simulink model "SimV8"  (R2024b)
settings: Solver=FixedStepAuto  StartTime=0.0  StopTime=10  RelTol=1e-3
model workspace (MAT data in the model file):
  Sig = Simulink.Signal
  Sig.Dimensions = -1
  Sig.DimensionsMode = 'auto'
  Sig.Complexity = 'auto'
  Sig.SampleTime = -1
  Sig.SamplingMode = 'auto'
  Sig.DataType = 'auto'
values from neighbouring files (symbols this model uses):
  CanaryAmplitude = 0.25    [ConfigData.sldd]
  CanaryCarrierFrequency = 20000.0    [ConfigData.sldd]
  CanaryDataRate = 100.0    [ConfigData.sldd]
  DataAmplitude = 0.1    [ConfigData.sldd]
  FmDecoderFrameSize = 128.0    [ConfigData.sldd]
  FmFrequencyDifferential = 400.0    [ConfigData.sldd]
  PreConvolveDownsample = 32.0    [ConfigData.sldd]
  SampleRate = 48000.0    [ConfigData.sldd]
  WalshCodeLength = 16.0    [ConfigData.sldd]
undefined symbols (not defined in the file or in its folder): FmFrequencyDataCache, ModulatedCanaryCachedCycle, WalshCodeCache
libraries: dspstat3 x4, simulink x3, dspfdesign x3, dspsnks4 x2, audiosources x2, commchan3 x1
settings Model: DataDictionary=ConfigData.sldd  PauseTimes=4.5  PacingRate=0.007100  Creator=calum  LastModifiedBy=calum
settings SolverCC: AllowMultiTaskInputOutput=on  PositivePriorityOrder=on  AutoInsertRateTranBlk=on
settings OptimizationCC: DefaultParameterBehavior=Inlined  InlineInvariantSignals=on  StateBitsets=on  DataBitsets=on  ZeroExternalMemoryAtStartup=off  ZeroInternalMemoryAtStartup=off  EfficientFloat2IntCast=on  SimCompilerOptimization=on  AccelVerboseBuild=on  MultiThreadedLoops=on
settings DebuggingCC: ReadBeforeWriteMsg=DisableAll  WriteAfterWriteMsg=DisableAll  WriteAfterReadMsg=DisableAll  MultiTaskDSMMsg=none  TasksWithSamePriorityMsg=none  IntegerOverflowMsg=none  IntegerSaturationMsg=none
settings HardwareCC: ProdBitPerLong=64  ProdLongLongMode=on  ProdHWDeviceType=AMD->x86-64 (Linux 64)  TargetBitPerLong=64  TargetBitPerPointer=64  TargetBitPerSizeT=64  TargetBitPerPtrDiffT=64  TargetLargestAtomicFloat=Float  TargetIntDivRoundTo=Zero  TargetEndianess=LittleEndian  TargetWordSize=64  TargetHWDeviceType=Intel->x86-64 (Linux 64)
settings ModelReferenceCC: UpdateModelReferenceTargets=IfOutOfDate  EnableParallelModelReferenceBuilds=on  ParallelModelReferenceMATLABWorkerInit=Copy Base Workspace
settings SFSimCC: SimUserLibraries=/home/calum/.local/matlab/2024b/bin/glnxa64/libmwdsp_halidesim.so  SFSimEcho=off  SimCtrlC=off  SimHardwareAcceleration=native  SimTargetLang=C++
settings RTWCC: GenerateReport=on  RTWUseSimCustomCode=on  CustomLibrary=/home/calum/.local/matlab/2024b/bin/glnxa64/libmwdsp_halidesim.so  BuildConfiguration=Faster Runs  LaunchReport=on  TargetLang=C++  CheckMdlBeforeBuild=Warning
settings CodeAppCC: MaxIdLength=95  MATLABSourceComments=on
settings GRTTargetCC: TargetLangStandard=C++17 (ISO)  MatFileLogging=off  CodeInterfacePackaging=C++ class  OptimizeReductions=on

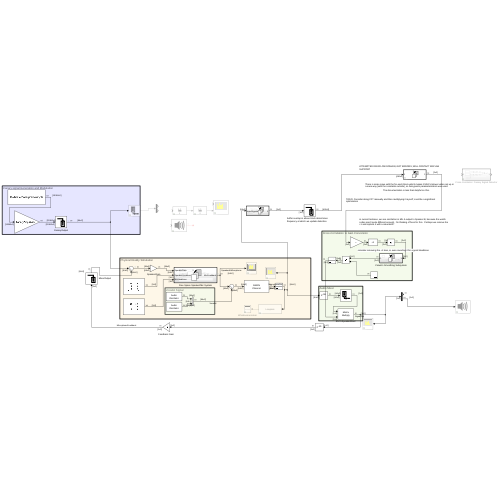
[thumbnail: Simulink's stored preview of the top-level diagram]
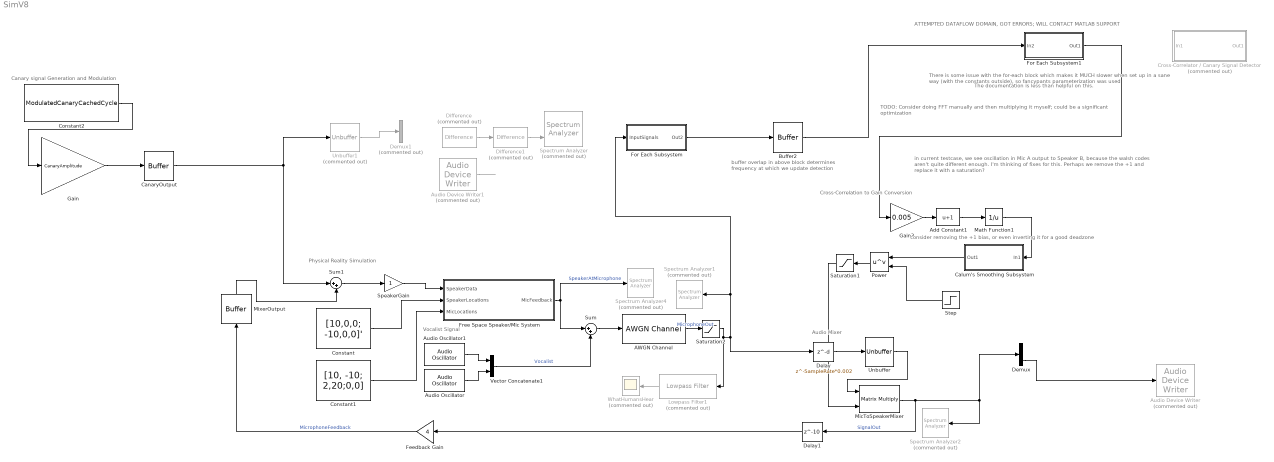
== system SimV8 ==
  note: The documentation is less than helpful on this.
  note: There is some issue with the for-each block which makes it MUCH slower when set up in a sane way (with the constants outside), so fancypants parameterization was used
  note: consider removing the +1 bias, or even inverting it for a good deadzone
  note: in current testcase, we see oscillation in Mic A output to Speaker B, because the walsh codes aren't quite different enough. I'm thinking of fixes for this. Perhaps we remove the +1 and replace it with a saturation?
  note: TODO: Consider doing FFT manually and then multiplying it myself; could be a significant optimization
  note: buffer overlap in above block determines frequency at which we update detection
  note: Canary signal Generation and Modulation
  note: Audio Mixer
  note: Physical Reality Simulation
  note: Vocalist Signal
  note: Cross-Correlation to Gain Conversion
  note: ATTEMPTED DATAFLOW DOMAIN, GOT ERRORS; WILL CONTACT MATLAB SUPPORT
  AWGN Channel : commchan3/AWGN Channel  LegacyMode=off  NoiseMethod="Signal to noise ratio  (SNR)"  noiseMode="Signal to noise ratio  (SNR)"  EbNo=10  EsNo=10  SNR=30  BitsPerSymbol=1  SignalPower=1  SamplesPerSymbol=1  SymbolPeriod=1  VarianceSource=Parameter  Variance=1  RandomStream=Global stream  Seed=67  SimulateUsing=Code generation
  Add Constant1 : Bias  Bias=1  SaturateOnIntegerOverflow=off
  Audio Device Writer : dspsnks4/Audio Device Writer  Commented=on  Driver=ALSA  Device=Default  InheritSampleRate=on  SampleRate=44100  BitDepth=16-bit integer  BufferSize=4096  NumBuffers=10  DefaultOutputChannelMapping=on  OutputChannelMapping=1:2  OutputNumUnderrunSamples=off  DriverIdx=8  DeviceWarnFlag=''
  Audio Device Writer1 : dspsnks4/Audio Device Writer  Commented=on  Driver=ALSA  Device=Default  InheritSampleRate=on  SampleRate=44100  BitDepth=16-bit integer  BufferSize=4096  NumBuffers=10  DefaultOutputChannelMapping=on  OutputChannelMapping=1:2  OutputNumUnderrunSamples=on  DriverIdx=8  DeviceWarnFlag=''
  Audio Oscillator : audiosources/Audio Oscillator  FrequencyPort=off  Frequency=200  AmplitudePort=off  Amplitude=DataAmplitude  DCOffsetPort=off  DCOffset=0  PhaseOffset=0  WidthPort=off  Width=1  DutyCyclePort=off  DutyCycle=0.5  SampsPerFrame=64  Fs=SampleRate  OutputDataType=double  SimulateUsing=Code generation
      settings: SignalType=sine
  Audio Oscillator1 : audiosources/Audio Oscillator  FrequencyPort=off  Frequency=400  AmplitudePort=off  Amplitude=DataAmplitude  DCOffsetPort=off  DCOffset=0  PhaseOffset=0  WidthPort=off  Width=1  DutyCyclePort=off  DutyCycle=0.5  SampsPerFrame=64  Fs=SampleRate  OutputDataType=double  SimulateUsing=Code generation
      settings: SignalType=sine
  Buffer2 : Buffer  N=ceil(SampleRate/32/CanaryDataRate*WalshCodeLength*2)+10  V=ceil(SampleRate/32/CanaryDataRate*WalshCodeLength*2)  OutputFrames=off
  Calum's Smoothing Subsystem : Subsystem  TreatAsAtomicUnit=on
  CanaryOutput : Buffer  OutputFrames=off
  Constant : Constant  Value="[10,0,0;  -10,0,0]'"
  Constant1 : Constant  Value=[10, -10; 2,20;0,0]
  Constant2 : Constant  Value=ModulatedCanaryCachedCycle
  "Cross-Correlator / Canary Signal Detector " : Subsystem  Commented=on  TreatAsAtomicUnit=on
  Delay : Delay  DelayLength=SampleRate*0.002  InitialCondition=0  InputProcessing=Columns as channels (frame based)  UseCircularBuffer=on
  Delay1 : Delay  DelayLength=10  InitialCondition=0  InputProcessing=Columns as channels (frame based)  UseCircularBuffer=on
  Demux : Demux  Outputs=2
  Demux1 : Demux  Commented=on  Outputs=2
  Difference : simulink/Discrete/Difference  Commented=on  ICPrevInput=0.0  OutMin=[]  OutMax=[]  OutDataType=fixdt(1, 16)  OutScaling=2^-10  DoSatur=off
  Difference1 : simulink/Discrete/Difference  Commented=on  ICPrevInput=0.0  OutMin=[]  OutMax=[]  OutDataType=fixdt(1, 16)  OutScaling=2^-10  DoSatur=off
  Feedback Gain : Gain  Gain=4
  For Each Subsystem : Subsystem  TreatAsAtomicUnit=on
  For Each Subsystem1 : Subsystem  TreatAsAtomicUnit=on  mask{CachedCode=WalshCodeCache}
      mask prompts: CachedCode "Walsh Codes"
      settings: RTWSystemCode=Inline
  Free Space Speaker/Mic System : Subsystem  TreatAsAtomicUnit=on
  Gain : Gain  Gain=CanaryAmplitude
  Gain3 : Gain  Gain=0.005
  Lowpass Filter1 : dspfdesign/Lowpass Filter  Commented=on  FilterType=FIR  DesignForMinimumOrder=on  FilterOrder=50  PassbandFrequency=CanaryCarrierFrequency-8000  StopbandFrequency=CanaryCarrierFrequency-1000  PassbandRipple=0.1  StopbandAttenuation=80  SampleRateMode=Specify on dialog  SampleRate=SampleRate  SimulateUsing=Code generation  roundingMode=Floor  coeffsDataTypeStr=fixdt(1,16)
  Math Function1 : Math  Operator=reciprocal
  MicToSpeakerMixer : Product  Multiplication=Matrix(*)
  MixerOutput : Buffer  OutputFrames=off
  Power : Math  Operator=pow
  Saturation1 : Saturate  UpperLimit=1  LowerLimit=0
  Saturation2 : Saturate  UpperLimit=1  LowerLimit=-1
  SpeakerGain : Gain
  Spectrum Analyzer : SpectrumAnalyzer  Commented=on  NumInputPorts=2  WindowPosition=[1.000000,38.000000,1920.000000,1003.000000,]  ScopeFrameLocation=window  SampleRate=44.1e3  PlotAsTwoSidedSpectrum=off  FrequencyScale=Log  WindowInvariantSamplesPerUpdate=on  StartFrequency=20  StopFrequency=20e3  YLimits=[-110.89284784388445,-17.687002082691375]  SelectedToolstripTab=spectrumAnalyzerToolstrip.estimationTab
      settings: OpenAtSimulationStart=off
  Spectrum Analyzer1 : SpectrumAnalyzer  Commented=on  WindowPosition=[1.000000,38.000000,1920.000000,1003.000000,]  ScopeFrameLocation=window  SampleRateSource=Property  SampleRate=SampleRate  PlotAsTwoSidedSpectrum=off  FrequencyScale=Log  FrequencySpan=Start and stop frequencies  StartFrequency=20  StopFrequency=20e3  YLimits=[-78.74086897,62.76889366]
  Spectrum Analyzer2 : SpectrumAnalyzer  Commented=on  WindowPosition=[1.000000,38.000000,1920.000000,1003.000000,]  ScopeFrameLocation=window  SampleRateSource=Property  SampleRate=SampleRate  PlotAsTwoSidedSpectrum=off  FrequencyScale=Log  FrequencySpan=Start and stop frequencies  StartFrequency=20  StopFrequency=20e3  YLimits=[-81.26361088,68.62221432]
  Spectrum Analyzer4 : SpectrumAnalyzer  Commented=on  WindowPosition=[1.000000,38.000000,1920.000000,1003.000000,]  ScopeFrameLocation=window  ViewType=Spectrum and spectrogram  SampleRateSource=Property  SampleRate=SampleRate  PlotAsTwoSidedSpectrum=off  FrequencyScale=Log  FrequencySpan=Start and stop frequencies  StartFrequency=20  StopFrequency=20e3  YLimits=[-136.03313301,69.13471038]  ColorLimits=[-136.03313301,69.13471038]
  Step : Step  Time=35  Before=5  After=0  SampleTime=1/(CanaryDataRate)
  Sum : Sum  Inputs=|++
  Sum1 : Sum  Inputs=|++
  Unbuffer : Unbuffer
  Unbuffer1 : Unbuffer  Commented=on
  Vector Concatenate1 : Concatenate  Mode=Multidimensional array  ConcatenateDimension=2
  WhatHumansHear : Scope  Commented=on
  wires:
  Sum1/1 -> SpeakerGain/1
  AWGN Channel/1 -> Saturation2/1  "MicrophoneOut"
  SpeakerGain/1 -> Free Space Speaker/Mic System/1(SpeakerData)
  Constant/1 -> Free Space Speaker/Mic System/2(SpeakerLocations)
  Constant1/1 -> Free Space Speaker/Mic System/3(MicLocations)
  Audio Oscillator1/1 -> Vector Concatenate1/1
  Audio Oscillator/1 -> Vector Concatenate1/2
  Add Constant1/1 -> Math Function1/1
  Gain3/1 -> Add Constant1/1
  Vector Concatenate1/1 -> Sum/2  "Vocalist"
  Free Space Speaker/Mic System/1(MicFeedback) -> Sum/1, Spectrum Analyzer4/1  "SpeakerAtMicrophone"
  Math Function1/1 -> Calum's Smoothing Subsystem/1(In1)
  MicToSpeakerMixer/1 -> Demux/1, Spectrum Analyzer2/1, Delay1/1  "SignalOut"
  Calum's Smoothing Subsystem/1(Out1) -> Power/1
  Step/1 -> Power/2
  Power/1 -> Saturation1/1
  Saturation1/1 -> MicToSpeakerMixer/2
  Sum/1 -> AWGN Channel/1
  Feedback Gain/1 -> MixerOutput/1  "MicrophoneFeedback"
  Lowpass Filter1/1 -> WhatHumansHear/1
  Buffer2/1 -> For Each Subsystem1/1(In2)
  For Each Subsystem1/1(Out1) -> Gain3/1
  For Each Subsystem/1(Out2) -> Buffer2/1
  Unbuffer/1 -> MicToSpeakerMixer/1
  Delay1/1 -> Feedback Gain/1
  Delay/1 -> Unbuffer/1
  MixerOutput/1 -> Sum1/2
  Constant2/1 -> Gain/1
  CanaryOutput/1 -> Unbuffer1/1, Sum1/1
  Unbuffer1/1 -> Demux1/1
  Audio Device Writer1/1 -> ?
  Difference1/1 -> Spectrum Analyzer/2
  Difference/1 -> Difference1/1
  Demux/2 -> Audio Device Writer/1
  Gain/1 -> CanaryOutput/1
  Saturation2/1 -> Lowpass Filter1/1, For Each Subsystem/1(InputSignals), Spectrum Analyzer1/1, Delay/1

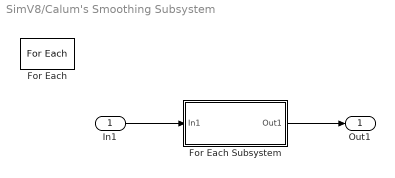
== system SimV8/Calum's Smoothing Subsystem ==
  In1 : Inport  Partition=on  PartitionDimension=1  PartitionWidth=1  PartitionOffset=0
  For Each : ForEach  DisableCoverage=on
  For Each Subsystem : Subsystem  TreatAsAtomicUnit=on
  Out1 : Outport  ConcatenationDimension=1
  wires:
  In1/1 -> For Each Subsystem/1(In1)
  For Each Subsystem/1(Out1) -> Out1/1

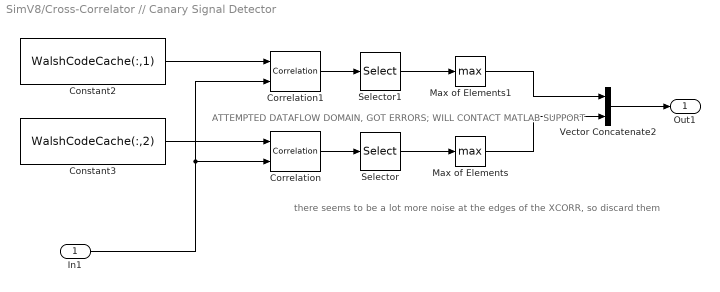
== system SimV8/Cross-Correlator // Canary Signal Detector  ==
  note: ATTEMPTED DATAFLOW DOMAIN, GOT ERRORS; WILL CONTACT MATLAB SUPPORT
  note: there seems to be a lot more noise at the edges of the XCORR, so discard them
  In1 : Inport
  Constant2 : Constant  Value=WalshCodeCache(:,1)  VectorParams1D=off
  Constant3 : Constant  Value=WalshCodeCache(:,2)  VectorParams1D=off
  Correlation : dspstat3/Correlation  domain=Fastest  roundingMode=Floor  overflowMode=off  outputDataTypeStr=Inherit: Same as accumulator  outputMin=[]  outputMax=[]  outputLastDataTypeStr=Inherit: Same as accumulator
  Correlation1 : dspstat3/Correlation  domain=Fastest  roundingMode=Floor  overflowMode=off  outputDataTypeStr=Inherit: Same as accumulator  outputMin=[]  outputMax=[]  outputLastDataTypeStr=Inherit: Same as accumulator
  Max of Elements : MinMax  Function=max  CollapseMode=Specified dimension
  Max of Elements1 : MinMax  Function=max  CollapseMode=Specified dimension
  Selector : Selector  NumberOfDimensions=2  InputPortWidth=3  IndexOptions=Index vector (dialog),Select all  Indices=[225 : 225+221],1  OutputSizes=1,1
  Selector1 : Selector  NumberOfDimensions=2  InputPortWidth=3  IndexOptions=Index vector (dialog),Select all  Indices=[225 : 225+221],1  OutputSizes=1,1
  Vector Concatenate2 : Concatenate  Mode=Multidimensional array
  Out1 : Outport
  wires:
  Constant2/1 -> Correlation1/1
  Selector/1 -> Max of Elements/1
  Constant3/1 -> Correlation/1
  Max of Elements1/1 -> Vector Concatenate2/1
  Max of Elements/1 -> Vector Concatenate2/2
  Correlation/1 -> Selector/1
  Correlation1/1 -> Selector1/1
  In1/1 -> Correlation/2, Correlation1/2
  Selector1/1 -> Max of Elements1/1
  Vector Concatenate2/1 -> Out1/1

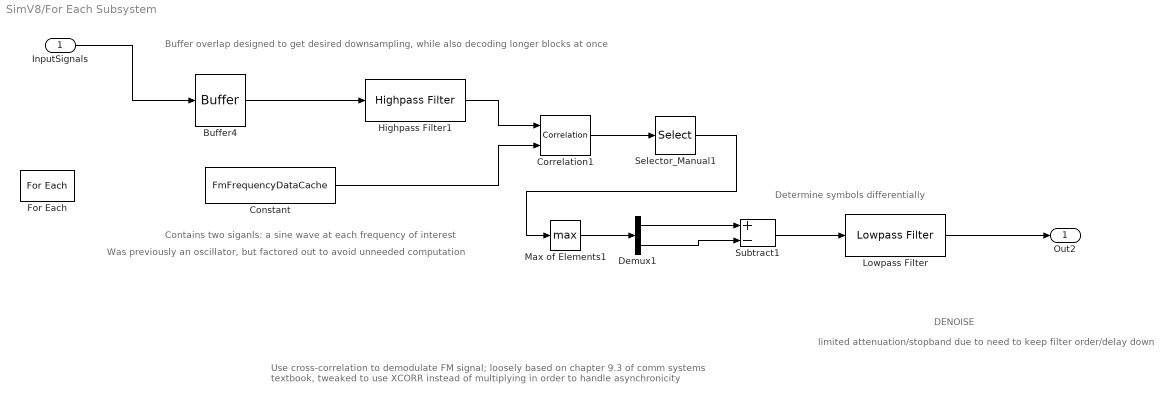
== system SimV8/For Each Subsystem ==
  note: Was previously an oscillator, but factored out to avoid unneeded computation
  note: Buffer overlap designed to get desired downsampling, while also decoding longer blocks at once
  note: Contains two siganls: a sine wave at each frequency of interest
  note: limited attenuation/stopband due to need to keep filter order/delay down
  note: DENOISE
  note: Use cross-correlation to demodulate FM signal; loosely based on chapter 9.3 of comm systems textbook, tweaked to use XCORR instead of multiplying in order to handle asynchronicity
  note: Determine symbols differentially
  InputSignals : Inport  Partition=on  PartitionDimension=2  PartitionWidth=1  PartitionOffset=0
  Buffer4 : Buffer  N=FmDecoderFrameSize  V=FmDecoderFrameSize-PreConvolveDownsample  OutputFrames=off
  Constant : Constant  Value=FmFrequencyDataCache
  Correlation1 : dspstat3/Correlation  domain=Fastest  roundingMode=Floor  overflowMode=off  outputDataTypeStr=Inherit: Same as accumulator  outputMin=[]  outputMax=[]  outputLastDataTypeStr=Inherit: Same as accumulator
  Demux1 : Demux  Outputs=2
  For Each : ForEach  DisableCoverage=on
  Highpass Filter1 : dspfdesign/Highpass Filter  FilterType=FIR  DesignForMinimumOrder=on  FilterOrder=50  StopbandFrequency=CanaryCarrierFrequency-FmFrequencyDifferential-CanaryDataRate*10  PassbandFrequency=CanaryCarrierFrequency-FmFrequencyDifferential-CanaryDataRate*2  StopbandAttenuation=80  PassbandRipple=1  SampleRateMode=Specify on dialog  SampleRate=SampleRate  SimulateUsing=Code generation  roundingMode=Floor  coeffsDataTypeStr=fixdt(1,16)
  Lowpass Filter : dspfdesign/Lowpass Filter  FilterType=FIR  DesignForMinimumOrder=on  FilterOrder=50  PassbandFrequency=CanaryDataRate*2  StopbandFrequency=CanaryDataRate*3  PassbandRipple=0.1  StopbandAttenuation=60  SampleRateMode=Specify on dialog  SampleRate=SampleRate/PreConvolveDownsample  SimulateUsing=Code generation  roundingMode=Floor  coeffsDataTypeStr=fixdt(1,16)
  Max of Elements1 : MinMax  Function=max  CollapseMode=Specified dimension
  Selector_Manual1 : Selector  NumberOfDimensions=2  InputPortWidth=3  IndexOptions=Starting index (dialog),Select all  Indices=FmDecoderFrameSize/2,1  OutputSizes=FmDecoderFrameSize,1
  Subtract1 : Sum  Inputs=+-
  Out2 : Outport  ConcatenationDimension=2
  wires:
  InputSignals/1 -> Buffer4/1
  Demux1/2 -> Subtract1/2
  Selector_Manual1/1 -> Max of Elements1/1
  Demux1/1 -> Subtract1/1
  Subtract1/1 -> Lowpass Filter/1
  Max of Elements1/1 -> Demux1/1
  Highpass Filter1/1 -> Correlation1/1
  Constant/1 -> Correlation1/2
  Buffer4/1 -> Highpass Filter1/1
  Correlation1/1 -> Selector_Manual1/1
  Lowpass Filter/1 -> Out2/1

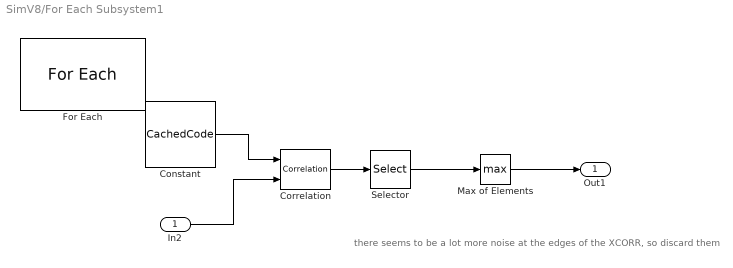
== system SimV8/For Each Subsystem1 ==
  note: there seems to be a lot more noise at the edges of the XCORR, so discard them
  In2 : Inport
  Constant : Constant  Value=CachedCode
  Correlation : dspstat3/Correlation  domain=Fastest  roundingMode=Floor  overflowMode=off  outputDataTypeStr=Inherit: Same as accumulator  outputMin=[]  outputMax=[]  outputLastDataTypeStr=Inherit: Same as accumulator
  For Each : ForEach  DisableCoverage=on  IterateSubsysMaskParameter=on  SubsysMaskParameterIterationDimension=2
  Max of Elements : MinMax  Function=max  CollapseMode=Specified dimension
  Selector : Selector  NumberOfDimensions=2  InputPortWidth=3  IndexOptions=Starting index (dialog),Select all  Indices=length(WalshCodeCache)/2+10,1  OutputSizes=ceil(SampleRate/32/CanaryDataRate*WalshCodeLength*2)-10,1
  Out1 : Outport  ConcatenationDimension=1
  wires:
  Correlation/1 -> Selector/1
  Selector/1 -> Max of Elements/1
  Constant/1 -> Correlation/1
  Max of Elements/1 -> Out1/1
  In2/1 -> Correlation/2

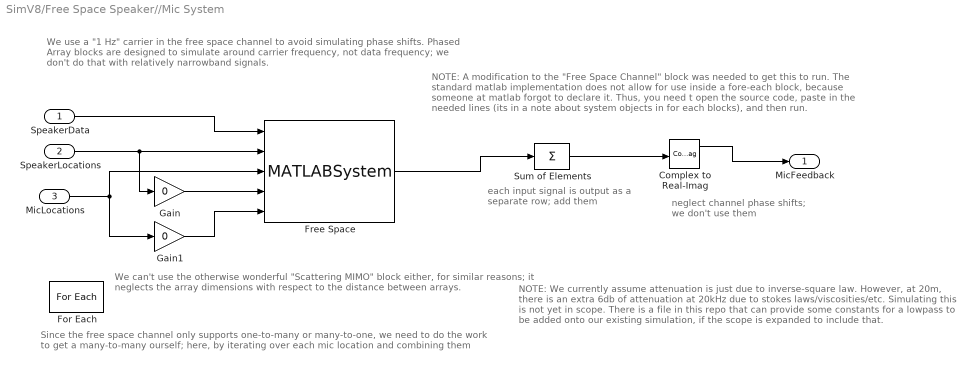
== system SimV8/Free Space Speaker//Mic System ==
  note: NOTE: We currently assume attenuation is just due to inverse-square law.
      | However, at 20m, there is an extra 6db of attenuation at 20kHz due to stokes laws/viscosities/etc.  Simulating this is not yet in scope.  There is a file in this repo that can provide some constants for a lowpass to be added onto our existing simulation, if the scope is expanded to include that.
  note: neglect channel phase
      | shifts; we don't use them
  note: each input signal is output as
      | a separate row; add them
  note: NOTE: A modification to the "Free Space Channel" block was needed to get
      | this to run.  The standard matlab implementation does not allow for use inside a fore-each block, because someone at matlab forgot to declare it.  Thus, you need t open the source code, paste in the needed lines (its in a note about system objects in for each blocks), and then run.
  note: Since the free space channel only supports one-to-many or many-to-one, we need to do the work to get a many-to-many ourself; here, by iterating over each mic location and combining them
  note: We can't use the otherwise wonderful "Scattering MIMO" block either, for similar reasons;
      | it neglects the array dimensions with respect to the distance between arrays.
  note: We use a "1 Hz" carrier in the free space channel to avoid simulating phase shifts.
      | Phased Array blocks are designed to simulate around carrier frequency, not data frequency; we don't do that
      | with relatively narrowband signals.
  SpeakerData : Inport
  SpeakerLocations : Inport  Port=2
  MicLocations : Inport  Port=3  Partition=on  PartitionDimension=2  PartitionWidth=1  PartitionOffset=0
  Complex to Real-Imag : ComplexToRealImag
  For Each : ForEach  DisableCoverage=on
  Free Space : MATLABSystem  System=FreeSpaceCalum  PropagationSpeed=SoundSpeed  OperatingFrequency=0.000001  TwoWayPropagation=off  SampleRateFromInputCheckbox=on  SampleRate=1e6  MaximumDistanceSource=Property  MaximumDistance=10e3  MaximumNumInputSamplesSource=Auto  MaximumNumInputSamples=100  SimulateUsing=Code generation
      settings: LibrarySourceBlock=phasedenvlib/Free Space
      mask Type: FreeSpaceCalum
      mask Display:
      | disp(['Free Space' char(10) 'Channel (Calum''s)']);
      | port_label('input',1,'X');
      | port_label('input',2,'Pos1');
      | port_label('input',3,'Pos2');
      | port_label('input',4,'Vel1');
      | port_label('input',5,'Vel2');
  Gain : Gain  Gain=0
  Gain1 : Gain  Gain=0
  Sum of Elements : Sum  Inputs=+  CollapseMode=Specified dimension  CollapseDim=2
  MicFeedback : Outport  ConcatenationDimension=2
  wires:
  SpeakerData/1 -> Free Space/1
  SpeakerLocations/1 -> Free Space/2, Gain/1
  Free Space/1 -> Sum of Elements/1
  Sum of Elements/1 -> Complex to Real-Imag/1
  Gain/1 -> Free Space/4
  Gain1/1 -> Free Space/5
  MicLocations/1 -> Gain1/1, Free Space/3
  Complex to Real-Imag/1 -> MicFeedback/1

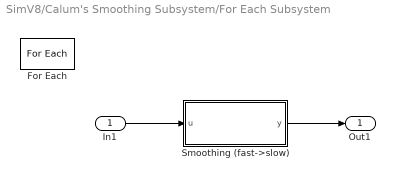
== system SimV8/Calum's Smoothing Subsystem/For Each Subsystem ==
  In1 : Inport  Partition=on  PartitionDimension=2  PartitionWidth=1  PartitionOffset=0
  For Each : ForEach  DisableCoverage=on
  Smoothing (fast->slow) : Subsystem  mask(Smoothing (fast->slow)){nSmooth=floor(SampleRate/CanaryDataRate/PreConvolveDownsample), h1=-1, smoothing0=1}
      mask prompts: nSmooth "physmod:simscape:couplers:SimscapeNetworkCouplersLib:NumberOfSamplesOverWhichToSmooth_MP"; h1 "physmod:simscape:couplers:SimscapeNetworkCouplersLib:PortUDiscreteSampleTimes_MP"; smoothing0 "physmod:simscape:couplers:SimscapeNetworkCouplersLib:InitialOutput_MP"
      mask help: physmod:simscape:couplers:SimscapeNetworkCouplersLib:Smoothingfastslow_MD
      mask Help: web([docroot '/simscape/ref/smoothingfastslow.html'])
      mask DialogControl nSmooth Prompt: Number of samples over which to smooth
      mask DialogControl h1 Prompt: Port u discrete sample time (s)
      mask DialogControl smoothing0 Prompt: Initial output
  Out1 : Outport  ConcatenationDimension=2
  wires:
  In1/1 -> Smoothing (fast->slow)/1(u)
  Smoothing (fast->slow)/1(y) -> Out1/1

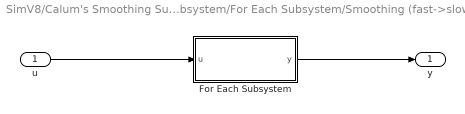
== system SimV8/Calum's Smoothing Subsystem/For Each Subsystem/Smoothing (fast->slow) ==
  u : Inport
  For Each Subsystem : Subsystem  TreatAsAtomicUnit=on
  y : Outport
  wires:
  For Each Subsystem/1(y) -> y/1
  u/1 -> For Each Subsystem/1(u)

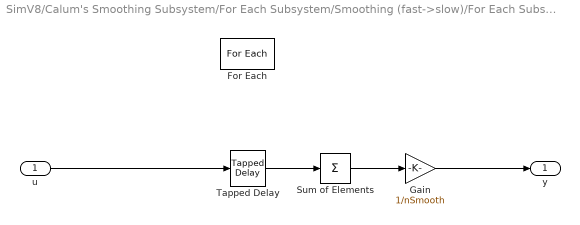
== system SimV8/Calum's Smoothing Subsystem/For Each Subsystem/Smoothing (fast->slow)/For Each Subsystem ==
  u : Inport  Partition=on  PartitionDimension=1  PartitionWidth=1  PartitionOffset=0
  For Each : ForEach  DisableCoverage=on
  Gain : Gain  Gain=1/nSmooth
  Sum of Elements : Sum  Inputs=+
  Tapped Delay : simulink/Discrete/Tapped Delay  vinit=mean(smoothing0)  samptime=h1  NumDelays=nSmooth  DelayOrder=Oldest  includeCurrent=off
  y : Outport  ConcatenationDimension=1
  wires:
  u/1 -> Tapped Delay/1
  Sum of Elements/1 -> Gain/1
  Tapped Delay/1 -> Sum of Elements/1
  Gain/1 -> y/1
